simulink model "SixDOFSim"  (R2020b)
settings: Solver=VariableStepAuto  StartTime=0.0  StopTime=20  RelTol=1e-3
values from neighbouring files (symbols this model uses):
  A = sys.A    [coupling_control.m]    (also in defineABC.m = [A_1 zeros(n/2,n/2);zeros(n/2,n/2) A_2]; implicit_linmod.m = -inv(E)*A_prime; nonlinear_6DOF.m = q_d*S*CA; nonlinear_model.m = q*S*CA)
  B = sys.B    [coupling_control.m]    (also in defineABC.m = [B_1, zeros(n/2,m/2);zeros(n/2,m/2), B_2]; implicit_linmod.m = -inv(E)*B_prime; normieren.m = Tx\B*Tu; steuerbarHautus.m)
  eta_max = 10*pi/180    (= 0.174532925199)    [SixDOFModel.m]
  eta_min = - 25*pi/180    (= -0.436332312999)    [SixDOFModel.m]
  I_inv = inv(I)    [initializeParameters.m]    (also in nonlinear_model6DOF.m = globalParameters.I_inv)
  K = place(A,B,ew_contr)    [SixDOFModel.m]
  latlon_init = [0;0]    [SixDOFModel.m]
  m = 9300    [OnePointOfMassModel.m]    (also in coupling_control.m = i-1; defineABC.m = size(B_1,2) + size(B_2,2); implicit_linmod.m = length(U_ap); initializeParameters.m = 120000)
  Omega_init = [0;0;0]    [SixDOFModel.m]
  P_e_init = [0;0;-h_init]    [SixDOFModel.m]
  Phi_init = [0;0;0]    [SixDOFModel.m]
  sigmaf_max = 10*pi/180    (= 0.174532925199)    [SixDOFModel.m]
  sigmaf_min = 0.5*pi/180    (= 0.00872664625997)    [SixDOFModel.m]
  U_ap = Z_ap(13:16)    [trimValues.m]
  U_test = U_ap    [SixDOFModel.m]
  V_init = [85;0;0]    [SixDOFModel.m]
  X_ap = 1.0e+03*[0.0907;0.0000;0.0005;0.0000;0.0000;0.0000;0.0000;0.0000;0.0000;1.0000]    [linearisierung.m]    (also in trimValues.m = Z_ap(1:12))
  X_init = X_ap    [SixDOFModel.m]
  xi_max = 25*pi/180    (= 0.436332312999)    [SixDOFModel.m]
  xi_min = - xi_max    (= -0.436332312999)    [SixDOFModel.m]
  zita_max = 30*pi/180    (= 0.523598775598)    [SixDOFModel.m]
  zita_min = - zita_max    (= -0.523598775598)    [SixDOFModel.m]
undefined symbols (not defined in the file or in its folder): Earth, nonlinear_6DOF, WGS84
libraries: aerolibfltsims x13, aerolibtransform2 x3, aerolibwind2 x1, aerolibatmos2 x1
settings Model: Creator=teteu  LastModifiedBy=teteu
settings SolverCC: ZeroCrossAlgorithm=Adaptive
settings DebuggingCC: IgnoredZcDiagnostic=none

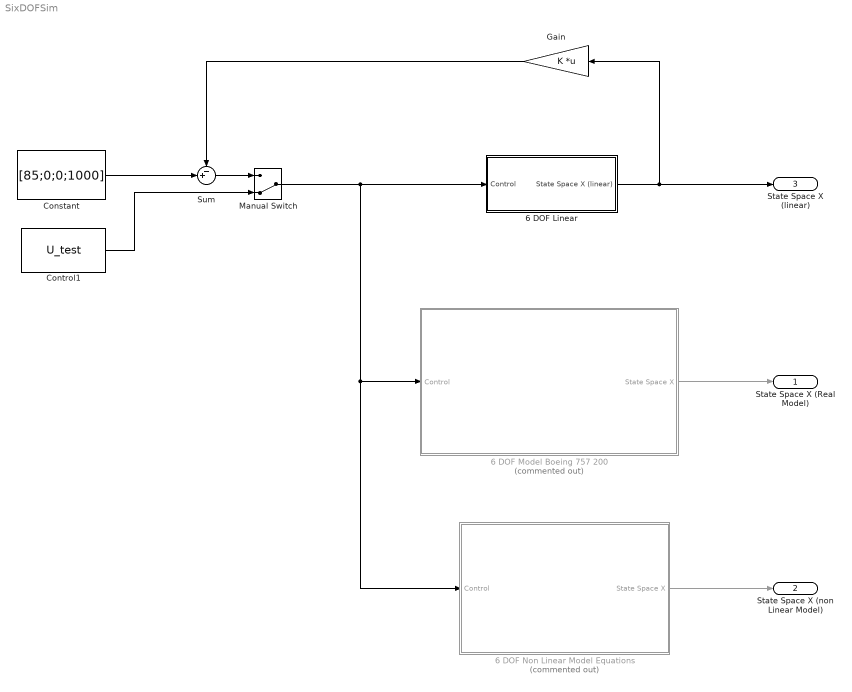
== system SixDOFSim ==
  6 DOF Linear : Subsystem
  6 DOF Model Boeing 757 200 : Subsystem  Commented=on
      mask Display: image('Eastern_Airlines_Boeing_757-225_N523EA_March_1990_DCW_4974892113-624x422.jpg'); % Use "Edit Image" on toolstrip to change.
  6 DOF Non Linear Model Equations : Subsystem  Commented=on
      mask Display: image('491461_1_En_8_Fig2_HTML.png');
  Constant : Constant  Value=[85;0;0;1000]
  Control1 : Constant  Value=U_test
  Gain : Gain  Gain=K  Multiplication=Matrix(K*u)
  Manual Switch : ManualSwitch  CurrentSetting=0
  Sum : Sum  Inputs=-+|
  State Space X (Real Model) : Outport
  State Space X (non Linear Model) : Outport  Port=2
  State Space X (linear) : Outport  Port=3
  wires:
  6 DOF Model Boeing 757 200/1(State Space X) -> State Space X (Real Model)/1
  Gain/1 -> Sum/1
  Constant/1 -> Sum/2
  Sum/1 -> Manual Switch/1
  Control1/1 -> Manual Switch/2
  Manual Switch/1 -> 6 DOF Linear/1(Control), 6 DOF Non Linear Model Equations/1(Control), 6 DOF Model Boeing 757 200/1(Control)
  6 DOF Linear/1(State Space X (linear)) -> Gain/1, State Space X (linear)/1
  6 DOF Non Linear Model Equations/1(State Space X) -> State Space X (non Linear Model)/1

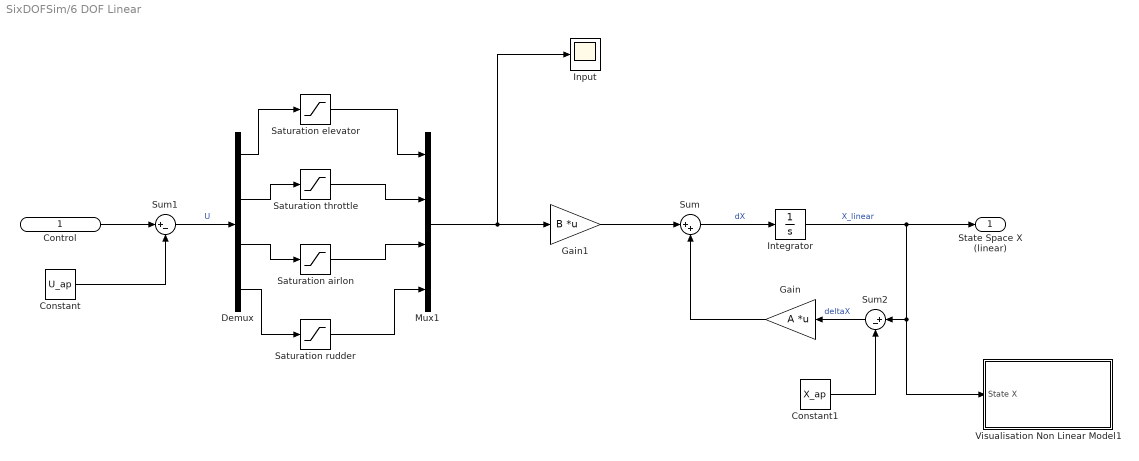
== system SixDOFSim/6 DOF Linear ==
  Control : Inport
  Constant : Constant  Value=U_ap
  Constant1 : Constant  Value=X_ap
  Demux : Demux
  Gain : Gain  Gain=A  Multiplication=Matrix(K*u)
  Gain1 : Gain  Gain=B  Multiplication=Matrix(K*u)
  Input : Scope
  Integrator : Integrator  InitialCondition=X_init
  Mux1 : Mux
  Saturation airlon : Saturate  UpperLimit=xi_max  LowerLimit=xi_min
  Saturation elevator : Saturate  UpperLimit=eta_max  LowerLimit=eta_min
  Saturation rudder : Saturate  UpperLimit=zita_max  LowerLimit=zita_min
  Saturation throttle : Saturate  UpperLimit=sigmaf_max  LowerLimit=sigmaf_min
  Sum : Sum  Inputs=|++
  Sum1 : Sum  Inputs=|+-
  Sum2 : Sum  Inputs=|+-
  Visualisation Non Linear Model1 : Subsystem
  State Space X (linear) : Outport
  wires:
  Gain1/1 -> Sum/1
  Mux1/1 -> Input/1, Gain1/1
  Sum/1 -> Integrator/1  "dX"
  Gain/1 -> Sum/2
  Demux/2 -> Saturation throttle/1
  Demux/3 -> Saturation airlon/1
  Demux/1 -> Saturation elevator/1
  Saturation elevator/1 -> Mux1/1
  Saturation throttle/1 -> Mux1/2
  Saturation airlon/1 -> Mux1/3
  Saturation rudder/1 -> Mux1/4
  Demux/4 -> Saturation rudder/1
  Control/1 -> Sum1/1
  Sum1/1 -> Demux/1  "U"
  Constant/1 -> Sum1/2
  Integrator/1 -> Visualisation Non Linear Model1/1(State X), Sum2/1, State Space X (linear)/1  "X_linear"
  Sum2/1 -> Gain/1  "deltaX"
  Constant1/1 -> Sum2/2

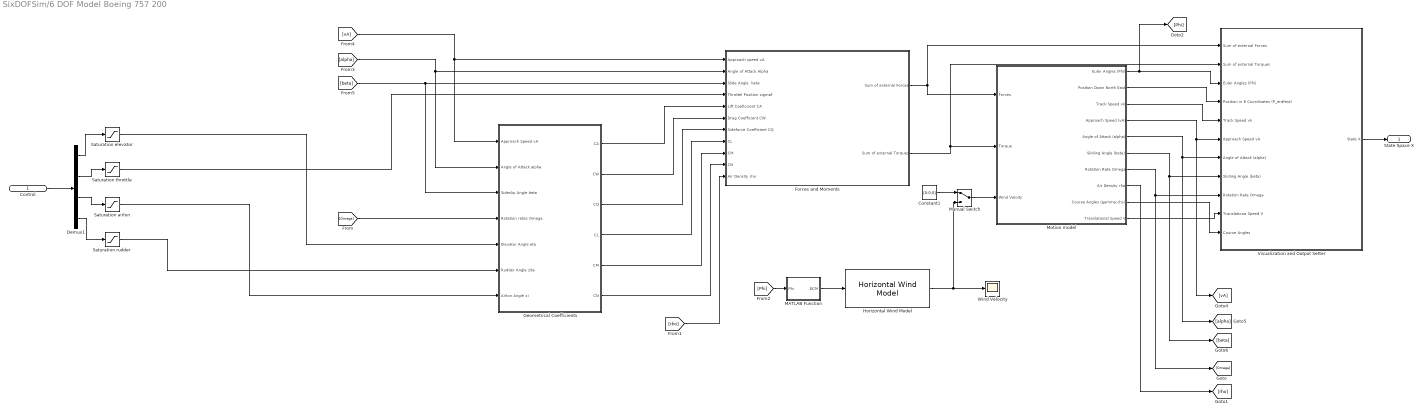
== system SixDOFSim/6 DOF Model Boeing 757 200 ==
  Control : Inport
  Constant1 : Constant  Value=[0;0;0]
  Demux1 : Demux
  Forces and Moments : Subsystem
  Geometrical Coefficients : Subsystem
  Horizontal Wind Model : aerolibwind2/Horizontal Wind Model  units=Metric (MKS)  Vw_source=Internal  Vwind=15  W_source=Internal  Wdeg=0
      settings: SourceProductBaseCode=AE
  MATLAB Function : MATLAB Function  TreatAsAtomicUnit=on
  Manual Switch : ManualSwitch
  "Motion model " : Subsystem
  Saturation airlon : Saturate  UpperLimit=xi_max  LowerLimit=xi_min
  Saturation elevator : Saturate  UpperLimit=eta_max  LowerLimit=eta_min
  Saturation rudder : Saturate  UpperLimit=zita_max  LowerLimit=zita_min
  Saturation throttle : Saturate  UpperLimit=sigmaf_max  LowerLimit=sigmaf_min
  Visualization and Output Setter : Subsystem
  Wind Velocity : Scope
  State Space X : Outport
  wires:
  "Motion model "/7(Rotation Rate Omega) -> [Omega], Visualization and Output Setter/9(Rotation Rate Omega)
  "Motion model "/3(Track Speed vk) -> Visualization and Output Setter/5(Track Speed vk)
  Visualization and Output Setter/1(State X) -> State Space X/1
  "Motion model "/6(Slidiing Angle (beta)) -> [beta], Visualization and Output Setter/8(Slidiing Angle (beta))
  Forces and Moments/2(Sum of external Torques) -> Visualization and Output Setter/2(Sum of external Torques), "Motion model "/2(Torque)
  [alpha] -> Geometrical Coefficients/2(Angle of Attack alpha), Forces and Moments/2(Angle of Attack Alpha)
  "Motion model "/4(Approach Speed (vA)) -> [vA], Visualization and Output Setter/6(Approach Speed vA)
  Geometrical Coefficients/4(CL) -> Forces and Moments/8(CL)
  Geometrical Coefficients/1(CA) -> Forces and Moments/5(Lift Coeficcient CA)
  Forces and Moments/1(Sum of external Forces) -> Visualization and Output Setter/1(Sum of external Forces), "Motion model "/1(Forces)
  "Motion model "/5(Angle of Attack (alpha)) -> [alpha], Visualization and Output Setter/7(Angle of Attack (alpha))
  "Motion model "/2(Position Down North East) -> Visualization and Output Setter/4(Position in E Coordinates (P_erdfest))
  "Motion model "/1(Euler Angles (Phi)) -> [Phi], Visualization and Output Setter/3(Euler Angles (Phi))
  [vA] -> Geometrical Coefficients/1(Approach Speed vA), Forces and Moments/1(Approach speed vA)
  Geometrical Coefficients/5(CM) -> Forces and Moments/9(CM)
  Saturation airlon/1 -> Geometrical Coefficients/7(Airlon Angle xi)
  [Omega] -> Geometrical Coefficients/4(Rotation rates Omega)
  Saturation throttle/1 -> Forces and Moments/4(Throttel Position sigmaf)
  [beta] -> Geometrical Coefficients/3(Sideslip Angle beta), Forces and Moments/3(Slide Angle  beta)
  Geometrical Coefficients/6(CN) -> Forces and Moments/10(CN)
  "Motion model "/8(Air Density rho) -> [rho]
  [rho] -> Forces and Moments/11(Air Density rho)
  Saturation elevator/1 -> Geometrical Coefficients/5(Elevator Angle eta)
  Saturation rudder/1 -> Geometrical Coefficients/6(Rudder Angle zita)
  Geometrical Coefficients/3(CQ) -> Forces and Moments/7(Sideforce Coefficient CQ)
  Geometrical Coefficients/2(CW) -> Forces and Moments/6(Drag Coefficient CW)
  MATLAB Function/1(DCM) -> Horizontal Wind Model/1
  Demux1/2 -> Saturation throttle/1
  Demux1/3 -> Saturation airlon/1
  Demux1/1 -> Saturation elevator/1
  Control/1 -> Demux1/1
  Demux1/4 -> Saturation rudder/1
  "Motion model "/9("Course Angles (gamma;chsi) ") -> Visualization and Output Setter/11("Course Angles ")
  "Motion model "/10(Translational Speed V) -> Visualization and Output Setter/10(Translationa Speed V)
  Horizontal Wind Model/1 -> Manual Switch/2, Wind Velocity/1
  Manual Switch/1 -> "Motion model "/3(Wind Veloity)
  Constant1/1 -> Manual Switch/1
  [Phi] -> MATLAB Function/1(Phi)

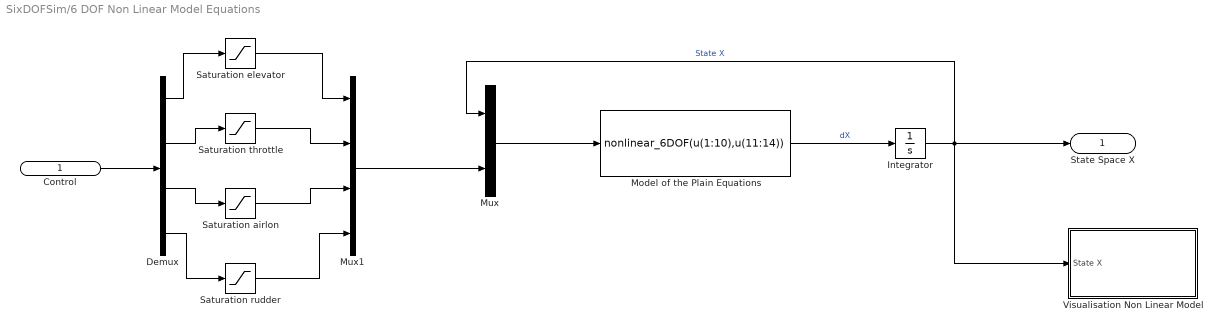
== system SixDOFSim/6 DOF Non Linear Model Equations ==
  Control : Inport
  Demux : Demux
  Integrator : Integrator  InitialCondition=X_init
  Model of the Plain Equations : MATLABFcn  MATLABFcn=nonlinear_6DOF(u(1:10),u(11:14))
  Mux : Mux  Inputs=2
  Mux1 : Mux
  Saturation airlon : Saturate  UpperLimit=xi_max  LowerLimit=xi_min
  Saturation elevator : Saturate  UpperLimit=eta_max  LowerLimit=eta_min
  Saturation rudder : Saturate  UpperLimit=zita_max  LowerLimit=zita_min
  Saturation throttle : Saturate  UpperLimit=sigmaf_max  LowerLimit=sigmaf_min
  Visualisation Non Linear Model : Subsystem
  State Space X : Outport
  wires:
  Model of the Plain Equations/1 -> Integrator/1  "dX"
  Integrator/1 -> State Space X/1, Visualisation Non Linear Model/1(State X), Mux/1  "State X"
  Mux/1 -> Model of the Plain Equations/1
  Demux/1 -> Saturation elevator/1
  Demux/2 -> Saturation throttle/1
  Demux/3 -> Saturation airlon/1
  Demux/4 -> Saturation rudder/1
  Saturation elevator/1 -> Mux1/1
  Saturation throttle/1 -> Mux1/2
  Saturation airlon/1 -> Mux1/3
  Saturation rudder/1 -> Mux1/4
  Mux1/1 -> Mux/2
  Control/1 -> Demux/1

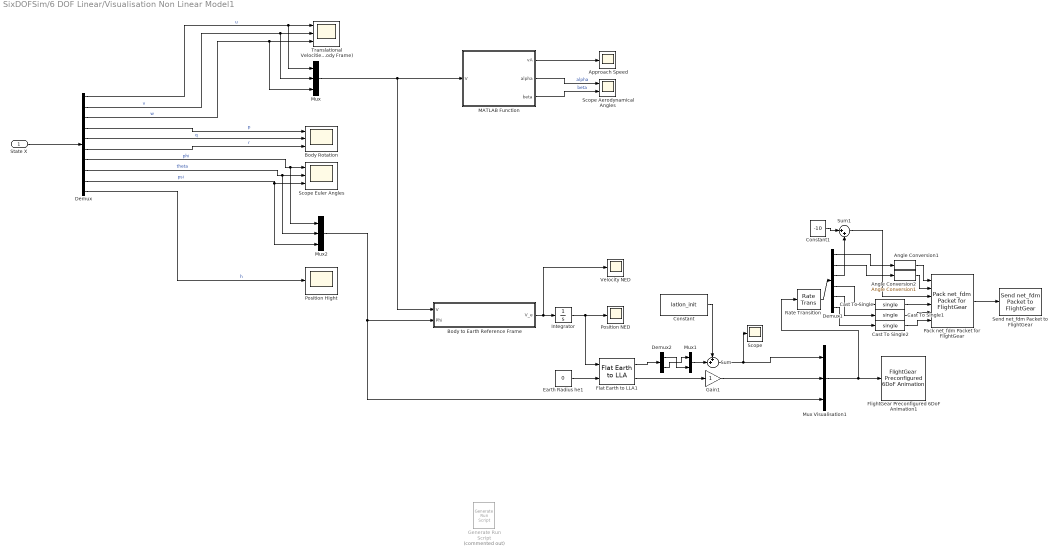
== system SixDOFSim/6 DOF Linear/Visualisation Non Linear Model1 ==
  State X : Inport
  Angle Conversion1 : aerolibfltsims/FlightGear Preconfigured 6DoF Animation/Angle Conversion1  SystemSampleTime=-1  VariantActivationTime=update diagram  Latency=0  AutoFrameSizeCalculation=off
      settings: SourceProductBaseCode=AE
  Angle Conversion2 : aerolibfltsims/FlightGear Preconfigured 6DoF Animation/Angle Conversion1  SystemSampleTime=-1  VariantActivationTime=update diagram  Latency=0  AutoFrameSizeCalculation=off
      settings: SourceProductBaseCode=AE
  Approach Speed : Scope
  Body Rotation : Scope  NumInputPorts=3
  "Body to Earth Reference Frame " : MATLAB Function  TreatAsAtomicUnit=on
  Cast To Single : DataTypeConversion  OutDataTypeStr=single
  Cast To Single1 : DataTypeConversion  OutDataTypeStr=single
  Cast To Single2 : DataTypeConversion  OutDataTypeStr=single
  Constant : Constant  Value=latlon_init
  Constant1 : Constant  Value=-10
  Demux : Demux  Outputs=10
  Demux1 : Demux  Outputs=6
  Demux2 : Demux  Outputs=2
  Earth Radius he1 : Constant  Value=0
  Flat Earth to LLA1 : aerolibtransform2/Flat Earth to LLA  units=Metric (MKS)  ptype=Earth (WGS84)  F=1/298.257223563  R=6378137  refPosPort=off  LL0=[0 10]  psi=0
  FlightGear Preconfigured 6DoF Animation1 : aerolibfltsims/FlightGear Preconfigured 6DoF Animation  xFlightGearVersion=v2019.1  DestinationIpAddress=127.0.0.1  DestinationPort=5502  SampleTime=1/30  packetVersion=24
  Gain1 : Gain
  Generate Run Script : aerolibfltsims/Generate Run Script  Commented=on  Architecture=Win64  dataFlow=Send  GeometryModelName=c172p  AirportId=KSFO  RunwayId=10L  InitialAltitude=7224  InitialHeading=113  OffsetDistance=4.72  OffsetAzimuth=0  InstallScenery=off  DisableShaders=on  OriginAddress=127.0.0.1  DestinationPort=5502  OriginPort=5505  LocalAddress=127.0.0.1  OutputFileName=runfg.bat  FlightGearBaseDirectory=D:\Flight Gear\FlightGear 2018.1.1
  Integrator : Integrator  InitialCondition=P_e_init
  MATLAB Function : MATLAB Function  TreatAsAtomicUnit=on
  Mux : Mux  Inputs=3
  Mux Visualisation1 : Mux  Inputs=3
  Mux1 : Mux  Inputs=2
  Mux2 : Mux  Inputs=3
  Pack net_fdm Packet for FlightGear : aerolibfltsims/Pack net_fdm Packet for FlightGear  FlightGearVersion=v2019.1  ShowPositionAttitudeInputs=on  ShowVelocityAccelerationInputs=off  ShowControlSurfacePositionInputs=off  ShowEngineFuelInputs=off  ShowLandingGearInputs=off  ShowEnvironmentInputs=off  SampleTime=1/30  packetVersion=24
      settings: SourceProductBaseCode=AE
  Position Hight : Scope
  Position NED : Scope
  Rate Transition : RateTransition  Integrity=off  Deterministic=off
  Scope : Scope
  Scope Aerodynamical Angles : Scope  NumInputPorts=2
  Scope Euler Angles : Scope  NumInputPorts=3
  Send net_fdm Packet to FlightGear : aerolibfltsims/Send net_fdm Packet to FlightGear  DestinationIpAddress=127.0.0.1  DestinationPort=5503  LocalIpPort=-1  varLen=off  SampleTime=1/30
      settings: SourceProductBaseCode=AE
  Sum : Sum  Inputs=++|
  Sum1 : Sum  Inputs=|++
  Translational Velocities (Body Frame) : Scope  NumInputPorts=3
  Velocity NED : Scope
  wires:
  State X/1 -> Demux/1
  Demux2/2 -> Mux1/1
  Flat Earth to LLA1/2 -> Gain1/1
  Gain1/1 -> Mux Visualisation1/2
  Mux Visualisation1/1 -> FlightGear Preconfigured 6DoF Animation1/1, Rate Transition/1
  Earth Radius he1/1 -> Flat Earth to LLA1/2
  Flat Earth to LLA1/1 -> Demux2/1
  Demux2/1 -> Mux1/2
  "Body to Earth Reference Frame "/1(V_e) -> Velocity NED/1, Integrator/1
  Integrator/1 -> Position NED/1, Flat Earth to LLA1/1
  Demux/1 -> Mux/1, Translational Velocities (Body Frame)/1  "u"
  Demux/2 -> Mux/2, Translational Velocities (Body Frame)/2  "v"
  Demux/3 -> Translational Velocities (Body Frame)/3, Mux/3  "w"
  Demux/4 -> Body Rotation/1  "p"
  Demux/5 -> Body Rotation/2  "q"
  Demux/6 -> Body Rotation/3  "r"
  Demux/7 -> Mux2/1, Scope Euler Angles/1  "phi"
  Demux/8 -> Mux2/2, Scope Euler Angles/2  "theta"
  Demux/9 -> Mux2/3, Scope Euler Angles/3  "psi"
  Demux/10 -> Position Hight/1  "h"
  Mux/1 -> MATLAB Function/1(V), "Body to Earth Reference Frame "/1(V)
  Mux2/1 -> "Body to Earth Reference Frame "/2(Phi), Mux Visualisation1/3
  MATLAB Function/1(vA) -> Approach Speed/1
  MATLAB Function/2(alpha) -> Scope Aerodynamical Angles/1  "alpha"
  MATLAB Function/3(beta) -> Scope Aerodynamical Angles/2  "beta"
  Mux1/1 -> Sum/2
  Sum/1 -> Scope/1, Mux Visualisation1/1
  Constant/1 -> Sum/1
  Pack net_fdm Packet for FlightGear/1 -> Send net_fdm Packet to FlightGear/1
  Angle Conversion1/1 -> Pack net_fdm Packet for FlightGear/1
  Angle Conversion2/1 -> Pack net_fdm Packet for FlightGear/2
  Cast To Single/1 -> Pack net_fdm Packet for FlightGear/4
  Cast To Single1/1 -> Pack net_fdm Packet for FlightGear/5
  Cast To Single2/1 -> Pack net_fdm Packet for FlightGear/6
  Demux1/2 -> Angle Conversion2/1
  Rate Transition/1 -> Demux1/1
  Demux1/1 -> Angle Conversion1/1
  Constant1/1 -> Sum1/1
  Demux1/3 -> Sum1/2
  Sum1/1 -> Pack net_fdm Packet for FlightGear/3
  Demux1/4 -> Cast To Single/1
  Demux1/5 -> Cast To Single1/1
  Demux1/6 -> Cast To Single2/1

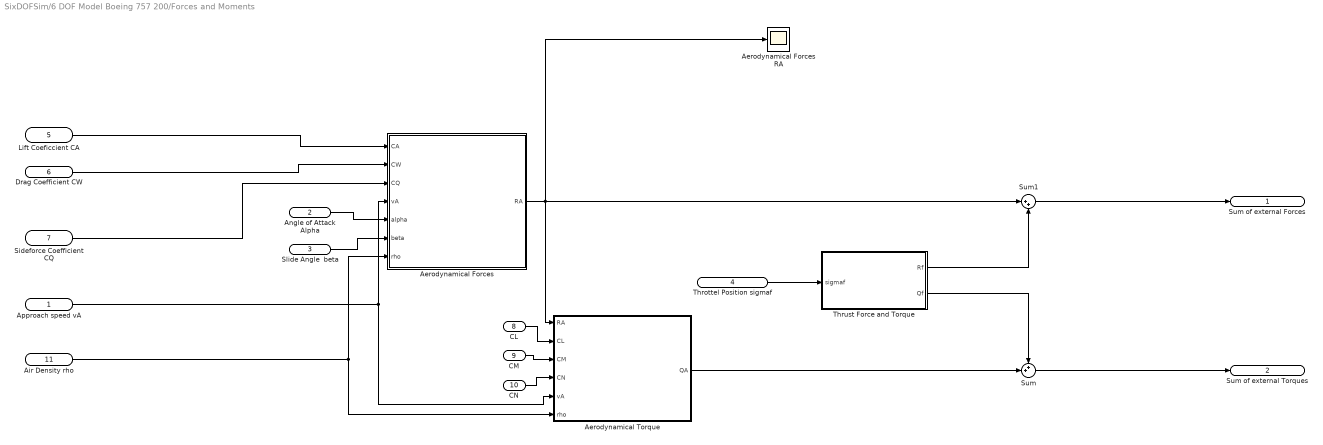
== system SixDOFSim/6 DOF Model Boeing 757 200/Forces and Moments ==
  Approach speed vA : Inport
  Angle of Attack Alpha : Inport  Port=2
  Slide Angle  beta : Inport  Port=3
  Throttel Position sigmaf : Inport  Port=4
  Lift Coeficcient CA : Inport  Port=5
  Drag Coefficient CW : Inport  Port=6
  Sideforce Coefficient CQ : Inport  Port=7
  CL : Inport  Port=8
  CM : Inport  Port=9
  CN : Inport  Port=10
  Air Density rho : Inport  Port=11
  Aerodynamical Forces : MATLAB Function  TreatAsAtomicUnit=on
  Aerodynamical Forces RA : Scope
  Aerodynamical Torque : MATLAB Function  TreatAsAtomicUnit=on
  Sum : Sum  Inputs=++|
  Sum1 : Sum  Inputs=|++
  Thrust Force and Torque : MATLAB Function  TreatAsAtomicUnit=on
  Sum of external Forces : Outport
  Sum of external Torques : Outport  Port=2
  wires:
  Aerodynamical Forces/1(RA) -> Aerodynamical Forces RA/1, Sum1/1, Aerodynamical Torque/1(RA)
  Aerodynamical Torque/1(QA) -> Sum/2
  Sum1/1 -> Sum of external Forces/1
  Sum/1 -> Sum of external Torques/1
  Throttel Position sigmaf/1 -> Thrust Force and Torque/1(sigmaf)
  Thrust Force and Torque/1(Rf) -> Sum1/2
  Thrust Force and Torque/2(Qf) -> Sum/1
  Angle of Attack Alpha/1 -> Aerodynamical Forces/5(alpha)
  Slide Angle  beta/1 -> Aerodynamical Forces/6(beta)
  Approach speed vA/1 -> Aerodynamical Forces/4(vA), Aerodynamical Torque/5(vA)
  Lift Coeficcient CA/1 -> Aerodynamical Forces/1(CA)
  Drag Coefficient CW/1 -> Aerodynamical Forces/2(CW)
  Sideforce Coefficient CQ/1 -> Aerodynamical Forces/3(CQ)
  CL/1 -> Aerodynamical Torque/2(CL)
  CM/1 -> Aerodynamical Torque/3(CM)
  CN/1 -> Aerodynamical Torque/4(CN)
  Air Density rho/1 -> Aerodynamical Forces/7(rho), Aerodynamical Torque/6(rho)

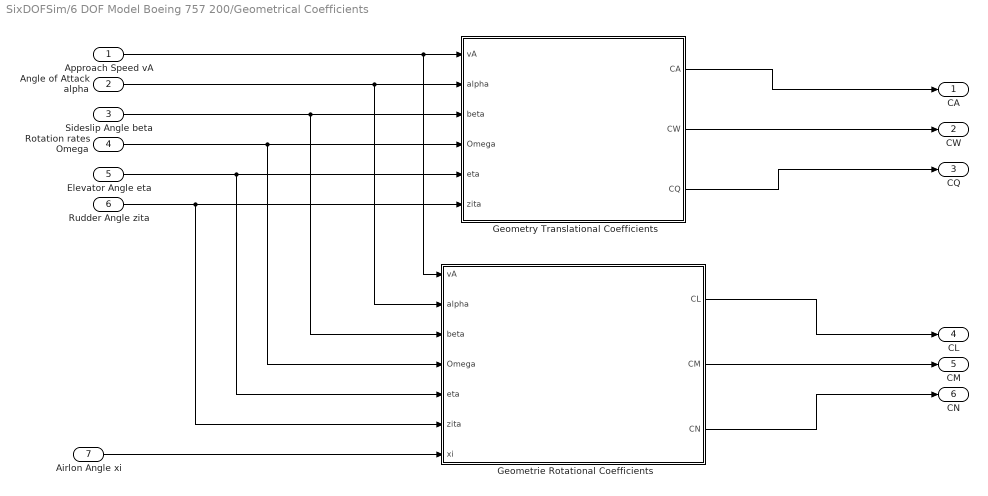
== system SixDOFSim/6 DOF Model Boeing 757 200/Geometrical Coefficients ==
  Approach Speed vA : Inport
  Angle of Attack alpha : Inport  Port=2
  Sideslip Angle beta : Inport  Port=3
  Rotation rates Omega : Inport  Port=4
  Elevator Angle eta : Inport  Port=5
  Rudder Angle zita : Inport  Port=6
  Airlon Angle xi : Inport  Port=7
  Geometrie Rotational Coefficients : MATLAB Function  TreatAsAtomicUnit=on
  Geometry Translational Coefficients : MATLAB Function  TreatAsAtomicUnit=on
  CA : Outport
  CW : Outport  Port=2
  CQ : Outport  Port=3
  CL : Outport  Port=4
  CM : Outport  Port=5
  CN : Outport  Port=6
  wires:
  Elevator Angle eta/1 -> Geometrie Rotational Coefficients/5(eta), Geometry Translational Coefficients/5(eta)
  Angle of Attack alpha/1 -> Geometrie Rotational Coefficients/2(alpha), Geometry Translational Coefficients/2(alpha)
  Geometrie Rotational Coefficients/1(CL) -> CL/1
  Geometry Translational Coefficients/3(CQ) -> CQ/1
  Geometrie Rotational Coefficients/3(CN) -> CN/1
  Approach Speed vA/1 -> Geometrie Rotational Coefficients/1(vA), Geometry Translational Coefficients/1(vA)
  Geometry Translational Coefficients/1(CA) -> CA/1
  Sideslip Angle beta/1 -> Geometrie Rotational Coefficients/3(beta), Geometry Translational Coefficients/3(beta)
  Rudder Angle zita/1 -> Geometrie Rotational Coefficients/6(zita), Geometry Translational Coefficients/6(zita)
  Geometry Translational Coefficients/2(CW) -> CW/1
  Rotation rates Omega/1 -> Geometrie Rotational Coefficients/4(Omega), Geometry Translational Coefficients/4(Omega)
  Geometrie Rotational Coefficients/2(CM) -> CM/1
  Airlon Angle xi/1 -> Geometrie Rotational Coefficients/7(xi)

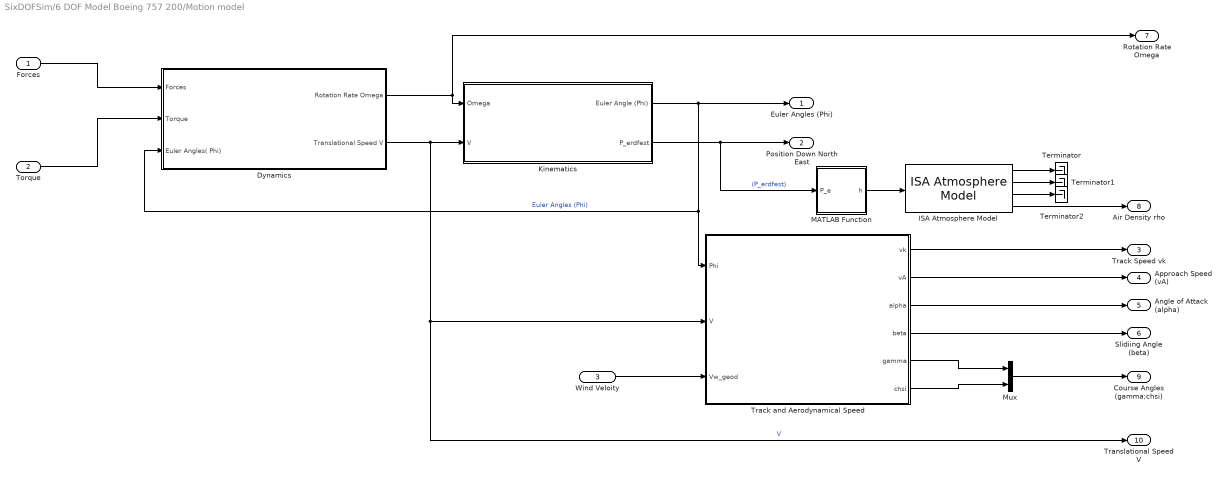
== system SixDOFSim/6 DOF Model Boeing 757 200/Motion model  ==
  Forces : Inport
  Torque : Inport  Port=2
  Wind Veloity : Inport  Port=3
  Dynamics : Subsystem
  ISA Atmosphere Model : aerolibatmos2/ISA Atmosphere Model  custom=off  g=9.80665  gamma=1.4  R=287.0531  L=0.0065  h_trop=11000  h_strat=20000  rho0=1.225  P0=101325  T0=288.15  h0=0
  Kinematics : Subsystem
  MATLAB Function : MATLAB Function  TreatAsAtomicUnit=on
  Mux : Mux  Inputs=2
  Terminator : Terminator
  Terminator1 : Terminator
  Terminator2 : Terminator
  Track and Aerodynamical Speed : MATLAB Function  TreatAsAtomicUnit=on
  Euler Angles (Phi) : Outport
  Position Down North East : Outport  Port=2
  Track Speed vk : Outport  Port=3
  Approach Speed (vA) : Outport  Port=4
  Angle of Attack (alpha) : Outport  Port=5
  Slidiing Angle (beta) : Outport  Port=6
  Rotation Rate Omega : Outport  Port=7
  Air Density rho : Outport  Port=8
  "Course Angles (gamma;chsi) " : Outport  Port=9
  Translational Speed V : Outport  Port=10
  wires:
  Torque/1 -> Dynamics/2(Torque)
  Kinematics/1(Euler Angle (Phi)) -> Track and Aerodynamical Speed/1(Phi), Dynamics/3(Euler Angles( Phi)), Euler Angles (Phi)/1  "Euler Angles (Phi)"
  Kinematics/2(P_erdfest) -> Position Down North East/1, MATLAB Function/1(P_e)  "(P_erdfest)"
  Dynamics/2(Translational Speed V) -> Kinematics/2(V), Translational Speed V/1, Track and Aerodynamical Speed/2(V)  "V"
  Forces/1 -> Dynamics/1(Forces)
  Dynamics/1(Rotation Rate Omega) -> Rotation Rate Omega/1, Kinematics/1(Omega)
  Wind Veloity/1 -> Track and Aerodynamical Speed/3(Vw_geod)
  MATLAB Function/1(h) -> ISA Atmosphere Model/1
  ISA Atmosphere Model/4 -> Air Density rho/1
  Track and Aerodynamical Speed/1(vk) -> Track Speed vk/1
  ISA Atmosphere Model/1 -> Terminator/1
  ISA Atmosphere Model/2 -> Terminator1/1
  ISA Atmosphere Model/3 -> Terminator2/1
  Track and Aerodynamical Speed/2(vA) -> Approach Speed (vA)/1
  Track and Aerodynamical Speed/3(alpha) -> Angle of Attack (alpha)/1
  Track and Aerodynamical Speed/4(beta) -> Slidiing Angle (beta)/1
  Mux/1 -> "Course Angles (gamma;chsi) "/1
  Track and Aerodynamical Speed/5(gamma) -> Mux/1
  Track and Aerodynamical Speed/6(chsi) -> Mux/2

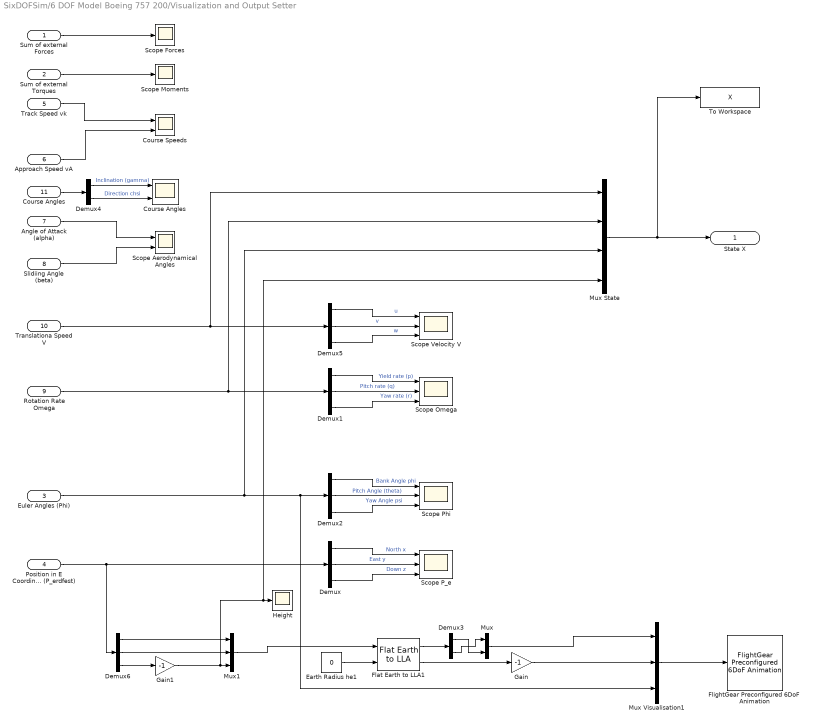
== system SixDOFSim/6 DOF Model Boeing 757 200/Visualization and Output Setter ==
  Sum of external Forces : Inport
  Sum of external Torques : Inport  Port=2
  Euler Angles (Phi) : Inport  Port=3
  Position in E Coordinates (P_erdfest) : Inport  Port=4
  Track Speed vk : Inport  Port=5
  Approach Speed vA : Inport  Port=6
  Angle of Attack (alpha) : Inport  Port=7
  Slidiing Angle (beta) : Inport  Port=8
  Rotation Rate Omega : Inport  Port=9
  Translationa Speed V : Inport  Port=10
  "Course Angles " : Inport  Port=11
  Course Angles : Scope  NumInputPorts=2
  Course Speeds : Scope  NumInputPorts=2
  Demux{,1..2,5..6} (5 alike) : Demux  Outputs=3
  Demux3 : Demux  Outputs=2
  Demux4 : Demux  Outputs=2
  Earth Radius he1 : Constant  Value=0
  Flat Earth to LLA1 : aerolibtransform2/Flat Earth to LLA  units=Metric (MKS)  ptype=Earth (WGS84)  F=1/298.257223563  R=6378137  refPosPort=off  LL0=[0 10]  psi=0
  FlightGear Preconfigured 6DoF Animation : aerolibfltsims/FlightGear Preconfigured 6DoF Animation  xFlightGearVersion=v2019.1  DestinationIpAddress=127.0.0.1  DestinationPort=5502  SampleTime=1/30  packetVersion=24
  Gain : Gain  Gain=-1
  Gain1 : Gain  Gain=-1
  Height : Scope
  Mux : Mux  Inputs=2
  Mux State : Mux
  Mux Visualisation1 : Mux  Inputs=3
  Mux1 : Mux  Inputs=3
  Scope Aerodynamical Angles : Scope  NumInputPorts=2
  Scope Forces : Scope
  Scope Moments : Scope
  Scope Omega : Scope  NumInputPorts=3
  Scope P_e : Scope  NumInputPorts=3
  Scope Phi : Scope  NumInputPorts=3
  Scope Velocity V : Scope  NumInputPorts=3
  To Workspace : ToWorkspace  VariableName=X  SaveFormat=Timeseries  SampleTime=-1
  State X : Outport
  wires:
  Mux State/1 -> To Workspace/1, State X/1
  Demux1/2 -> Scope Omega/2  "Pitch rate (q)"
  Demux2/2 -> Scope Phi/2  "Pitch Angle (theta)"
  Demux1/3 -> Scope Omega/3  "Yaw rate (r)"
  Demux1/1 -> Scope Omega/1  "Yield rate (p)"
  Demux2/1 -> Scope Phi/1  "Bank Angle phi"
  Demux/1 -> Scope P_e/1  "North x"
  Demux/2 -> Scope P_e/2  "East y"
  Demux/3 -> Scope P_e/3  "Down z"
  Demux2/3 -> Scope Phi/3  "Yaw Angle psi"
  Demux3/1 -> Mux/2
  Demux3/2 -> Mux/1
  Mux Visualisation1/1 -> FlightGear Preconfigured 6DoF Animation/1
  Flat Earth to LLA1/1 -> Demux3/1
  Earth Radius he1/1 -> Flat Earth to LLA1/2
  Mux/1 -> Mux Visualisation1/1
  Track Speed vk/1 -> Course Speeds/1
  Approach Speed vA/1 -> Course Speeds/2
  Sum of external Forces/1 -> Scope Forces/1
  Sum of external Torques/1 -> Scope Moments/1
  Demux4/1 -> Course Angles/1  "Inclination (gamma)"
  Demux4/2 -> Course Angles/2  "Direction chsi"
  "Course Angles "/1 -> Demux4/1
  Angle of Attack (alpha)/1 -> Scope Aerodynamical Angles/1
  Slidiing Angle (beta)/1 -> Scope Aerodynamical Angles/2
  Position in E Coordinates (P_erdfest)/1 -> Demux6/1, Demux/1
  Flat Earth to LLA1/2 -> Gain/1
  Gain/1 -> Mux Visualisation1/2
  Euler Angles (Phi)/1 -> Mux Visualisation1/3, Demux2/1, Mux State/3
  Rotation Rate Omega/1 -> Demux1/1, Mux State/2
  Demux5/3 -> Scope Velocity V/3  "w"
  Demux5/1 -> Scope Velocity V/1  "u"
  Demux5/2 -> Scope Velocity V/2  "v"
  Translationa Speed V/1 -> Demux5/1, Mux State/1
  Demux6/3 -> Gain1/1
  Gain1/1 -> Mux State/4, Height/1, Mux1/3
  Demux6/1 -> Mux1/1
  Demux6/2 -> Mux1/2
  Mux1/1 -> Flat Earth to LLA1/1

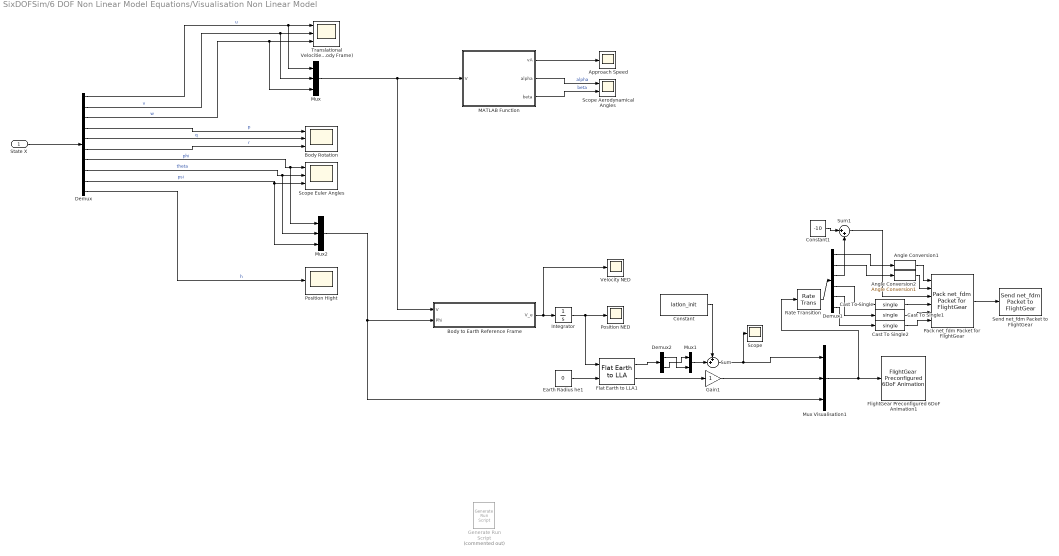
== system SixDOFSim/6 DOF Non Linear Model Equations/Visualisation Non Linear Model ==
  State X : Inport
  Angle Conversion1 : aerolibfltsims/FlightGear Preconfigured 6DoF Animation/Angle Conversion1  SystemSampleTime=-1  VariantActivationTime=update diagram  Latency=0  AutoFrameSizeCalculation=off
      settings: SourceProductBaseCode=AE
  Angle Conversion2 : aerolibfltsims/FlightGear Preconfigured 6DoF Animation/Angle Conversion1  SystemSampleTime=-1  VariantActivationTime=update diagram  Latency=0  AutoFrameSizeCalculation=off
      settings: SourceProductBaseCode=AE
  Approach Speed : Scope
  Body Rotation : Scope  NumInputPorts=3
  "Body to Earth Reference Frame " : MATLAB Function  TreatAsAtomicUnit=on
  Cast To Single : DataTypeConversion  OutDataTypeStr=single
  Cast To Single1 : DataTypeConversion  OutDataTypeStr=single
  Cast To Single2 : DataTypeConversion  OutDataTypeStr=single
  Constant : Constant  Value=latlon_init
  Constant1 : Constant  Value=-10
  Demux : Demux  Outputs=10
  Demux1 : Demux  Outputs=6
  Demux2 : Demux  Outputs=2
  Earth Radius he1 : Constant  Value=0
  Flat Earth to LLA1 : aerolibtransform2/Flat Earth to LLA  units=Metric (MKS)  ptype=Earth (WGS84)  F=1/298.257223563  R=6378137  refPosPort=off  LL0=[0 10]  psi=0
  FlightGear Preconfigured 6DoF Animation1 : aerolibfltsims/FlightGear Preconfigured 6DoF Animation  xFlightGearVersion=v2019.1  DestinationIpAddress=127.0.0.1  DestinationPort=5502  SampleTime=1/30  packetVersion=24
  Gain1 : Gain
  Generate Run Script : aerolibfltsims/Generate Run Script  Commented=on  Architecture=Win64  dataFlow=Send  GeometryModelName=c172p  AirportId=KSFO  RunwayId=10L  InitialAltitude=7224  InitialHeading=113  OffsetDistance=4.72  OffsetAzimuth=0  InstallScenery=off  DisableShaders=on  OriginAddress=127.0.0.1  DestinationPort=5502  OriginPort=5505  LocalAddress=127.0.0.1  OutputFileName=runfg.bat  FlightGearBaseDirectory=D:\Flight Gear\FlightGear 2018.1.1
  Integrator : Integrator  InitialCondition=P_e_init
  MATLAB Function : MATLAB Function  TreatAsAtomicUnit=on
  Mux : Mux  Inputs=3
  Mux Visualisation1 : Mux  Inputs=3
  Mux1 : Mux  Inputs=2
  Mux2 : Mux  Inputs=3
  Pack net_fdm Packet for FlightGear : aerolibfltsims/Pack net_fdm Packet for FlightGear  FlightGearVersion=v2019.1  ShowPositionAttitudeInputs=on  ShowVelocityAccelerationInputs=off  ShowControlSurfacePositionInputs=off  ShowEngineFuelInputs=off  ShowLandingGearInputs=off  ShowEnvironmentInputs=off  SampleTime=1/30  packetVersion=24
      settings: SourceProductBaseCode=AE
  Position Hight : Scope
  Position NED : Scope
  Rate Transition : RateTransition  Integrity=off  Deterministic=off
  Scope : Scope
  Scope Aerodynamical Angles : Scope  NumInputPorts=2
  Scope Euler Angles : Scope  NumInputPorts=3
  Send net_fdm Packet to FlightGear : aerolibfltsims/Send net_fdm Packet to FlightGear  DestinationIpAddress=127.0.0.1  DestinationPort=5503  LocalIpPort=-1  varLen=off  SampleTime=1/30
      settings: SourceProductBaseCode=AE
  Sum : Sum  Inputs=++|
  Sum1 : Sum  Inputs=|++
  Translational Velocities (Body Frame) : Scope  NumInputPorts=3
  Velocity NED : Scope
  wires:
  State X/1 -> Demux/1
  Demux2/2 -> Mux1/1
  Flat Earth to LLA1/2 -> Gain1/1
  Gain1/1 -> Mux Visualisation1/2
  Mux Visualisation1/1 -> FlightGear Preconfigured 6DoF Animation1/1, Rate Transition/1
  Earth Radius he1/1 -> Flat Earth to LLA1/2
  Flat Earth to LLA1/1 -> Demux2/1
  Demux2/1 -> Mux1/2
  "Body to Earth Reference Frame "/1(V_e) -> Velocity NED/1, Integrator/1
  Integrator/1 -> Position NED/1, Flat Earth to LLA1/1
  Demux/1 -> Mux/1, Translational Velocities (Body Frame)/1  "u"
  Demux/2 -> Mux/2, Translational Velocities (Body Frame)/2  "v"
  Demux/3 -> Translational Velocities (Body Frame)/3, Mux/3  "w"
  Demux/4 -> Body Rotation/1  "p"
  Demux/5 -> Body Rotation/2  "q"
  Demux/6 -> Body Rotation/3  "r"
  Demux/7 -> Mux2/1, Scope Euler Angles/1  "phi"
  Demux/8 -> Mux2/2, Scope Euler Angles/2  "theta"
  Demux/9 -> Mux2/3, Scope Euler Angles/3  "psi"
  Demux/10 -> Position Hight/1  "h"
  Mux/1 -> MATLAB Function/1(V), "Body to Earth Reference Frame "/1(V)
  Mux2/1 -> "Body to Earth Reference Frame "/2(Phi), Mux Visualisation1/3
  MATLAB Function/1(vA) -> Approach Speed/1
  MATLAB Function/2(alpha) -> Scope Aerodynamical Angles/1  "alpha"
  MATLAB Function/3(beta) -> Scope Aerodynamical Angles/2  "beta"
  Mux1/1 -> Sum/2
  Sum/1 -> Scope/1, Mux Visualisation1/1
  Constant/1 -> Sum/1
  Pack net_fdm Packet for FlightGear/1 -> Send net_fdm Packet to FlightGear/1
  Angle Conversion1/1 -> Pack net_fdm Packet for FlightGear/1
  Angle Conversion2/1 -> Pack net_fdm Packet for FlightGear/2
  Cast To Single/1 -> Pack net_fdm Packet for FlightGear/4
  Cast To Single1/1 -> Pack net_fdm Packet for FlightGear/5
  Cast To Single2/1 -> Pack net_fdm Packet for FlightGear/6
  Demux1/2 -> Angle Conversion2/1
  Rate Transition/1 -> Demux1/1
  Demux1/1 -> Angle Conversion1/1
  Constant1/1 -> Sum1/1
  Demux1/3 -> Sum1/2
  Sum1/1 -> Pack net_fdm Packet for FlightGear/3
  Demux1/4 -> Cast To Single/1
  Demux1/5 -> Cast To Single1/1
  Demux1/6 -> Cast To Single2/1

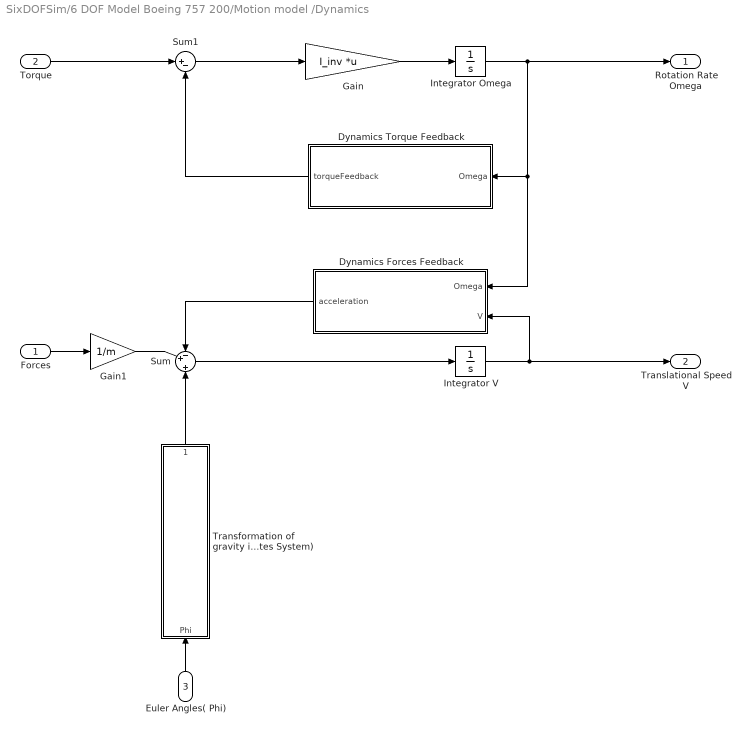
== system SixDOFSim/6 DOF Model Boeing 757 200/Motion model /Dynamics ==
  Forces : Inport
  Torque : Inport  Port=2
  Euler Angles( Phi) : Inport  Port=3
  Dynamics Forces Feedback : MATLAB Function  TreatAsAtomicUnit=on
  Dynamics Torque Feedback : MATLAB Function  TreatAsAtomicUnit=on
  Gain : Gain  Gain=I_inv  Multiplication=Matrix(K*u) (u vector)
  Gain1 : Gain  Gain=1/m
  Integrator Omega : Integrator  InitialCondition=Omega_init
  Integrator V : Integrator  InitialCondition=V_init
  Sum : Sum  Inputs=-+|+
  Sum1 : Sum  Inputs=|+-
  Transformation of gravity in (Körperfestes System) : MATLAB Function  TreatAsAtomicUnit=on
  Rotation Rate Omega : Outport
  Translational Speed V : Outport  Port=2
  wires:
  Euler Angles( Phi)/1 -> Transformation of gravity in (Körperfestes System)/1(Phi)
  Transformation of gravity in (Körperfestes System)/1(gravityAcceleration) -> Sum/3
  Forces/1 -> Gain1/1
  Sum/1 -> Integrator V/1
  Integrator V/1 -> Translational Speed V/1, Dynamics Forces Feedback/2(V)
  Gain1/1 -> Sum/2
  Dynamics Forces Feedback/1(acceleration) -> Sum/1
  Torque/1 -> Sum1/1
  Sum1/1 -> Gain/1
  Gain/1 -> Integrator Omega/1
  Integrator Omega/1 -> Dynamics Forces Feedback/1(Omega), Dynamics Torque Feedback/1(Omega), Rotation Rate Omega/1
  Dynamics Torque Feedback/1(torqueFeedback) -> Sum1/2

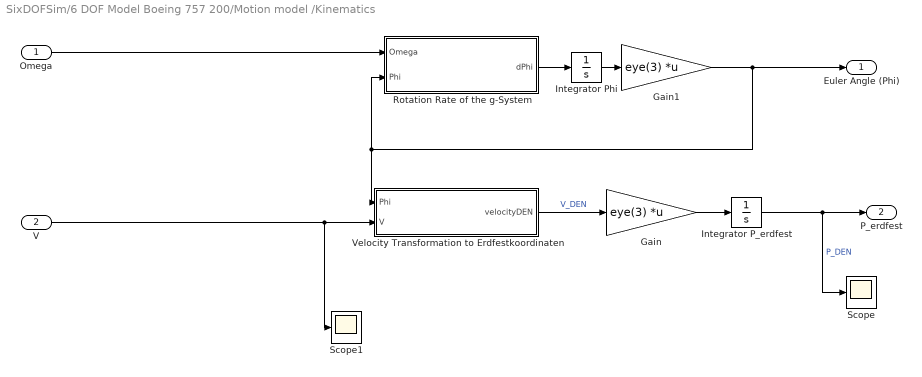
== system SixDOFSim/6 DOF Model Boeing 757 200/Motion model /Kinematics ==
  Omega : Inport
  V : Inport  Port=2
  Gain : Gain  Gain=eye(3)  Multiplication=Matrix(K*u) (u vector)
  Gain1 : Gain  Gain=eye(3)  Multiplication=Matrix(K*u) (u vector)
  Integrator P_erdfest : Integrator  InitialCondition=P_e_init
  Integrator Phi : Integrator  InitialCondition=Phi_init
  Rotation Rate of the g-System : MATLAB Function  TreatAsAtomicUnit=on
  Scope : Scope
  Scope1 : Scope
  Velocity Transformation to Erdfestkoordinaten : MATLAB Function  TreatAsAtomicUnit=on
  Euler Angle (Phi) : Outport
  P_erdfest : Outport  Port=2
  wires:
  Integrator P_erdfest/1 -> Scope/1, P_erdfest/1  "P_DEN"
  Velocity Transformation to Erdfestkoordinaten/1(velocityDEN) -> Gain/1  "V_DEN"
  V/1 -> Scope1/1, Velocity Transformation to Erdfestkoordinaten/2(V)
  Rotation Rate of the g-System/1(dPhi) -> Integrator Phi/1
  Gain/1 -> Integrator P_erdfest/1
  Omega/1 -> Rotation Rate of the g-System/1(Omega)
  Integrator Phi/1 -> Gain1/1
  Gain1/1 -> Rotation Rate of the g-System/2(Phi), Velocity Transformation to Erdfestkoordinaten/1(Phi), Euler Angle (Phi)/1

== matlab function SixDOFSim/6 DOF Model Boeing 757 200/Forces and Moments/Aerodynamical Torque ==
  data: RA input; CL input; QA output; CM input; CN input; vA input; globalParameters parameter; rho input
function QA = getAerodynTorque(RA,CL,CM,CN, vA, globalParameters,rho)
% h = P_e(3); %Height [m]
% [~,~,~,rho] = atmosisa(h); %Air density 
%Aircraft Parameters
b = globalParameters.b;
%rho = globalParameters.rho;
c = globalParameters.c;
S = globalParameters.S;
P_centerGravity = globalParameters.P_centerGravity;
P_aerodynCenter = globalParameters.P_aerodynCenter;
q_d = 0.5*vA^2*rho; %Dynamic Preassure


QA_aerodynCenter = q_d*S*[0.5*b*CL;c*CM;0.5*b*CN];
QA = QA_aerodynCenter + vecToMat(P_centerGravity- P_aerodynCenter)*RA;

== matlab function SixDOFSim/6 DOF Model Boeing 757 200/Forces and Moments/Thrust Force and Torque ==
  data: sigmaf input; Rf output; globalParameters parameter; Qf output
function [Rf,Qf] = thrust(sigmaf,globalParameters)
%Get Thrus Force Rf and Thrust Moment Qf
%sigmaf: Throttle Position [rad]
P_thrust =globalParameters.P_thrust;
i_f =globalParameters.i_f;
F_max = globalParameters.Fmax;

F_res = F_max*sigmaf; %Resultant Force Absolute Value
Rf = F_res*[cos(i_f);0;sin(i_f)]; %Thrust Force 
P_thrust_tilde = vecToMat(P_thrust);
Qf = P_thrust_tilde*Rf; %Thrust Moment

== matlab function SixDOFSim/6 DOF Model Boeing 757 200/Motion model /Dynamics/Dynamics Forces Feedback ==
  data: Omega input; V input; acceleration output; globalParameters parameter
function acceleration = accelerationFeedback(Omega,V,globalParameters)
Omega_e_tilde = globalParameters.Omega_e_tilde;
Omega_tilde = vecToMat(Omega);
acceleration = (Omega_tilde + Omega_e_tilde)*V;

== matlab function SixDOFSim/6 DOF Model Boeing 757 200/Motion model /Dynamics/Dynamics Torque Feedback ==
  data: Omega input; torqueFeedback output; globalParameters parameter
function torqueFeedback = getTorqueFeedback(Omega,globalParameters)
I = globalParameters.I;
Omega_tilde = vecToMat(Omega);
help = Omega_tilde*I;
torqueFeedback = help*Omega;

== matlab function SixDOFSim/6 DOF Model Boeing 757 200/Motion model /Dynamics/Transformation of gravity in (Körperfestes System) ==
  data: Phi input; gravityAcceleration output; g parameter
function gravityAcceleration = Tfg(Phi,g)
G_geod = [0;0;g]; %Graviation vector in geodetic ref. Frame
Tfg = coordTransfMatrix(Phi(1),1)*coordTransfMatrix(Phi(2),2)*coordTransfMatrix(Phi(3),3); % Transformation Matrix goedetic --> body reference Frame
gravityAcceleration = Tfg*G_geod;

== matlab function SixDOFSim/6 DOF Model Boeing 757 200/Motion model /Kinematics/Rotation Rate of the g-System ==
  data: Omega input; dPhi output; Phi input
function dPhi = J(Omega,Phi)
%Rotation rate of the g-system depending on the euler angles
%Phi: euler Angles
%Omega_ diff = Omega-Omega_g
%dPhi: Rotaion Speed considering the rotation rate of the geodathic system
phi = Phi(1);
theta = Phi(2);
J = 1/cos(theta)*[cos(theta) sin(phi)*sin(theta) cos(phi)*sin(theta) ;0 cos(phi)*cos(theta) -sin(phi)*cos(theta);0 sin(phi) cos(phi)]; %Rotation rate matrix
dPhi = J*Omega;

== matlab function SixDOFSim/6 DOF Model Boeing 757 200/Motion model /Kinematics/Velocity Transformation to Erdfestkoordinaten ==
  data: Phi input; V input; velocityDEN output
function velocityDEN = Tgf(Phi,V)
%Converts the velocity from Körper to Erdfest Koordinaten
%Phi: Vector w. Euler Angles
% P_erdfest: Position Vector 
phi = Phi(1);
theta = Phi(2);
psi = Phi(3);
Tfg =  coordTransfMatrix(phi,1)*coordTransfMatrix(theta,2)*coordTransfMatrix(psi,3); % Transformation Matrix goedetic --> body reference Frame
Tgf = Tfg';%Transformation to North East Down
velocityDEN = Tgf*V;

== matlab function SixDOFSim/6 DOF Model Boeing 757 200/Motion model /MATLAB Function ==
  data: P_e input; h output
function h = getHeight(P_e)
h = - P_e(3);

== matlab function SixDOFSim/6 DOF Model Boeing 757 200/Motion model /Track and Aerodynamical Speed ==
  data: Phi input; V input; vk output; vA output; alpha output; beta output; Vw_geod input; gamma output; chsi output
function [vk,vA,alpha,beta,gamma,chsi] = getTrackAndAero(Phi,V,Vw_geod)
%Get The Track Speed, the Approach Speed, the inclinational angle ,
%the Azimuth angle, the angle of attack and the Sliding angle from the
%Speed from the Translational Velocity. 
Tfg = coordTransfMatrix(Phi(1),1)*coordTransfMatrix(Phi(2),2)*coordTransfMatrix(Phi(3),3); % Transformation Matrix goedetic --> body reference Frame
Tgf = Tfg';
Vk = Tgf*V; %Track Velocity
vk = sqrt(Vk(1)^2+Vk(2)^2+Vk(3)^2); %Track Speed [m/s]
gamma = -asin(Vk(3)/vk); %Inclination Angle [rad]
chsi = atan2(Vk(2),Vk(1));
Vw = Tfg*Vw_geod;
VA = V - Vw; %Approach Speed
vA = sqrt(VA(1)^2+VA(2)^2+VA(3)^2); %Approach Speed [m/s]
alpha = atan(VA(3)/VA(1)); % Angle of attck [m/s]
beta = asin(VA(2)/vA);
% dvA = (VA(1)*dV(1) + VA(2)*dV(2) +VA(3)*dV(3))/(vA); %Derivative of the Approach Speed
% dalpha = (dV(3)*VA(1)-dV(1)*VA(3))/(VA(1)^2+VA(1)*VA(3)); %Derivative of Angle of Attack
% dbeta = (dV(2)*vA -dvA*VA(2))/(vA*sqrt(vA^2-VA(2)^2)); %Derivative of Sideslip Angle

== matlab function SixDOFSim/6 DOF Model Boeing 757 200/Geometrical Coefficients/Geometrie Rotational Coefficients ==
  data: vA input; alpha input; beta input; Omega input; eta input; zita input; globalParameters parameter; xi input; CL output; CM output; CN output
function [CL,CM,CN] = torqueGeometricCoefficient(vA,alpha,beta,Omega,eta,zita, globalParameters,xi)
%eta = Höheruderwinkel (elevator) [rad]
%zita = Seitenruderwinkel (ruder) [rad]
%xi = Querruderwinkel (Airlon) [rad]
%Global Parameters
lt = globalParameters.lt;
S = globalParameters.S;
St = globalParameters.St;
c = globalParameters.c;
alpha_L0 = -11.5*pi/180;
gradient_alpha_epsolon = 0.25;
epsolon = gradient_alpha_epsolon*(alpha - alpha_L0); %Downwash [rad]
%Moments Coefficients
N = [-1.4*beta;-0.59-3.1*(St*lt/(c*S))*(alpha-epsolon);(1-alpha*(180/(15*pi)))*beta]; %Static Moments Effects
Jakobi_CM_X = (c/vA)*[-11,    0,           5;
                      0,-4.03*St*lt^2/(S*c^2),0;
                      1.7,          0   , -11.5];
Jakobi_CM_U = [-0.6, 0, 0.22;
               0,    -3.1*St*lt/(S*c),0;
               0, 0, -0.63];      % Dependence of Control Variables
           
C_torque = N + Jakobi_CM_X*Omega + Jakobi_CM_U*[xi;eta;zita];
CL = C_torque(1);
CM = C_torque(2);
CN = C_torque(3);

== matlab function SixDOFSim/6 DOF Model Boeing 757 200/Geometrical Coefficients/Geometry Translational Coefficients ==
  data: vA input; alpha input; CA output; beta input; Omega input; globalParameters parameter; CW output; CQ output; eta input; zita input
function [CA,CW,CQ] = forceGeometryCoefficients(vA,alpha,beta,Omega,globalParameters,eta,zita)
%eta = Höheruderwinkel (elevator) [rad]
%zita = Seitenruderwinkel (ruder) [rad]
%Global Parameters
lt = globalParameters.lt;
S = globalParameters.S;
St = globalParameters.St;
% Rotration rates [rad/s]
q = Omega(2); %Nickrate (Pitch Rate)
%Constants Coefficients
grad_alpha = 5.5;
alpha_L0 = -11.5*pi/180;
gradient_alpha_epsolon = 0.25;
gradient_CQ_Cbeta = -1.6;
gradientCQ_Czita = 0.24;
CW0 = 0.13;
kappa = 0.07;
a3 = -768.5;
a2 = 609.2;
a1 = -155.2;
a0 = 15.212;
%Forces Coefficients
if alpha <=14.5*pi/180
     
     CA_F = grad_alpha*(alpha -alpha_L0);
else
     CA_F = a3*alpha^.3+a2*alpha^.2+a1*alpha +a0;% Lift Coefficient without the Control Aereas
end
epsolon = gradient_alpha_epsolon*(alpha - alpha_L0); %Downwash [rad]
alpha_t = alpha - epsolon + eta +1.3*q*lt/vA; %Angle of Attack of the Tail [rad]
CA_H = 3.1*(St/S)*alpha_t; %Lift Coefficient of the Control Aereas (Elevator-Tail)
CA = CA_F + CA_H; %Total Lift Coefficient
CW = CW0 + kappa*(5.5*alpha + 0.654)^2; %Drag Coefficient
CQ = gradient_CQ_Cbeta*beta + gradientCQ_Czita*zita;

== matlab function SixDOFSim/6 DOF Non Linear Model Equations/Visualisation Non Linear Model/Body to Earth Reference Frame  ==
  data: V input; Phi input; V_e output
function V_e = getEarthPosition(V,Phi)

Tfg = coordTransfMatrix(Phi(1),1)*coordTransfMatrix(Phi(2),2)*coordTransfMatrix(Phi(3),3); % Transformation Matrix goedetic --> body reference Frame
Tgf = Tfg';
V_e = Tgf*V;
V_e(3) =  V_e(3);

== matlab function SixDOFSim/6 DOF Non Linear Model Equations/Visualisation Non Linear Model/MATLAB Function ==
  data: V input; vA output; alpha output; beta output
function [vA,alpha,beta] = getAerodynamical(V)
u = V(1);
v = V(2);
w = V(3);
vA = sqrt(u^2+v^2+w^2);
alpha = atan2(w,u);
beta = asin(v/vA);

== matlab function SixDOFSim/6 DOF Model Boeing 757 200/MATLAB Function ==
  data: Phi input; DCM output
function DCM = getTfg(Phi)

DCM = coordTransfMatrix(Phi(1),1)*coordTransfMatrix(Phi(2),2)*coordTransfMatrix(Phi(3),3); % Transformation Matrix goedetic --> body reference Frame

== matlab function SixDOFSim/6 DOF Linear/Visualisation Non Linear Model1/Body to Earth Reference Frame  ==
  data: V input; Phi input; V_e output
function V_e = getEarthPosition(V,Phi)

Tfg = coordTransfMatrix(Phi(1),1)*coordTransfMatrix(Phi(2),2)*coordTransfMatrix(Phi(3),3); % Transformation Matrix goedetic --> body reference Frame
Tgf = Tfg';
V_e = Tgf*V;
V_e(3) =  V_e(3);

== matlab function SixDOFSim/6 DOF Linear/Visualisation Non Linear Model1/MATLAB Function ==
  data: V input; vA output; alpha output; beta output
function [vA,alpha,beta] = getAerodynamical(V)
u = V(1);
v = V(2);
w = V(3);
vA = sqrt(u^2+v^2+w^2);
alpha = atan2(w,u);
beta = asin(v/vA);

== matlab function SixDOFSim/6 DOF Model Boeing 757 200/Forces and Moments/Aerodynamical Forces ==
  data: CA input; RA output; CW input; CQ input; vA input; alpha input; beta input; rho input; globalParameters parameter
function RA = getAerodynForces(CA,CW,CQ,vA, alpha, beta, rho,globalParameters)
%[~,~,~,rho] = atmosisa(h); %Air density 
q_d = 0.5*vA^2*rho; %Dynamic Preassure
S = globalParameters.S ;


A = q_d*S*CA; %Lift Force [N]
W = q_d*S*CW; %Air Resistance [N]
Q = q_d*S*CQ; %Transverse Force [N]

Tfa = coordTransfMatrix(alpha,2)*coordTransfMatrix(-beta,3); %Transformation Matrix Aerodynamics -> Körperfest

RA_a =[-W;Q;-A];
RA = Tfa*RA_a;
